simulink model "Practica8_Simulink"  (R2024a)
settings: Solver=VariableStepAuto  StartTime=0.0  StopTime=10.0  RelTol=1e-3
InitFcn:
  | R = 2;
  | Kt = 0.01;
  | b = 0.0012;
  | L = 0.023;
  | Ke = 0.01;
  | J = 0.001;
  | Va = 5;
settings Model: Creator=Manuel  LastModifiedBy=Manuel

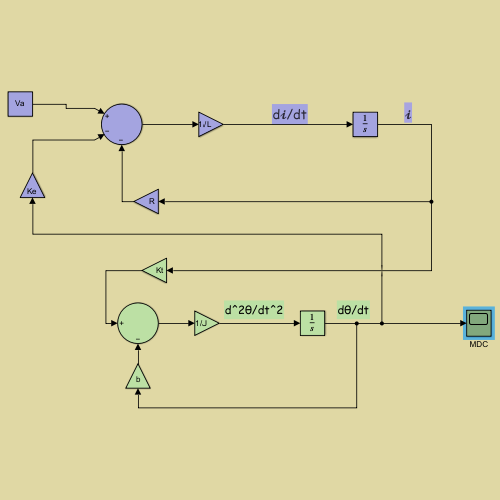
[thumbnail: Simulink's stored preview of the top-level diagram]
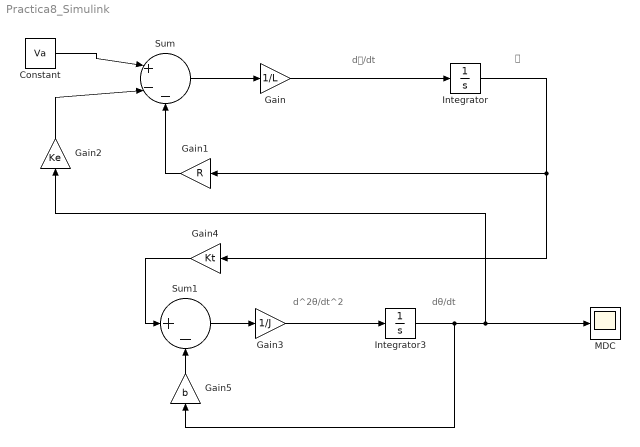
== system Practica8_Simulink ==
  note: 𝓲
  note: d𝓲/dt
  note: dθ/dt
  note: d^2θ/dt^2
  Constant : Constant  Value=Va
  Gain : Gain  Gain=1/L
  Gain1 : Gain  Gain=R
  Gain2 : Gain  Gain=Ke
  Gain3 : Gain  Gain=1/J
  Gain4 : Gain  Gain=Kt
  Gain5 : Gain  Gain=b
  Integrator : Integrator
  Integrator3 : Integrator
  MDC : Scope
  Sum : Sum  Inputs=|+--
  Sum1 : Sum  Inputs=|+-
  wires:
  Integrator/1 -> Gain4/1, Gain1/1
  Gain/1 -> Integrator/1
  Sum/1 -> Gain/1
  Gain2/1 -> Sum/2
  Gain1/1 -> Sum/3
  Integrator3/1 -> MDC/1, Gain2/1, Gain5/1
  Gain3/1 -> Integrator3/1
  Gain4/1 -> Sum1/1
  Sum1/1 -> Gain3/1
  Gain5/1 -> Sum1/2
  Constant/1 -> Sum/1
